simulink model "dk_luc"  (R2016a)
settings: Solver=ode45  StartTime=0.0  StopTime=322  RelTol=1e-3
settings Model: Creator=Trinh Hoang Minh  LastModifiedBy=Nam Nguyen
settings DataIOCC: LimitDataPoints=on  SaveFormat=Array  SignalLoggingSaveFormat=ModelDataLogs
settings OptimizationCC: ExpressionDepthLimit=2147483647
settings DebuggingCC: UnderspecifiedInitializationDetection=Classic  MergeDetectMultiDrivingBlocksExec=none  SolverPrmCheckMsg=warning  FcnCallInpInsideContextMsg=EnableAllAsWarning  StateNameClashWarn=warning
settings HardwareCC: ProdBitPerPointer=32  ProdLargestAtomicFloat=None  ProdIntDivRoundTo=Undefined  ProdEndianess=Unspecified  ProdWordSize=32  ProdHWDeviceType=32-bit Generic
settings ModelReferenceCC: PropagateSignalLabelsOutOfModel=off
settings ConfigComp: CovModelRefEnable=Off  CovSFcnEnable=off

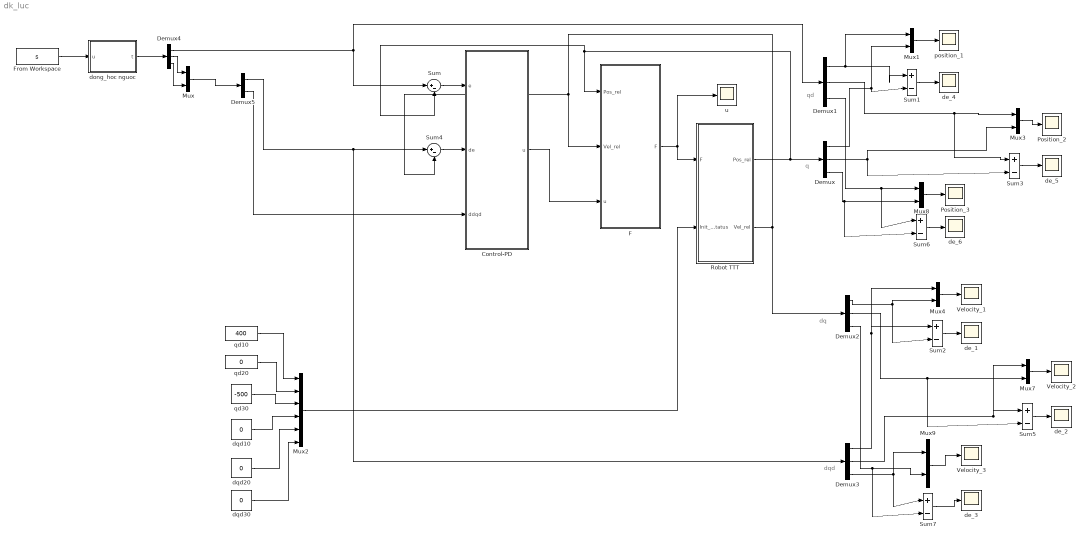
== system dk_luc ==
  note: q
  note: dq
  note: qd
  note: dqd
  Control-PD : Subsystem
  Demux{,1..4} (5 alike) : Demux  Outputs=3
  Demux5 : Demux  Outputs=2
  F : Subsystem
  From Workspace : FromWorkspace  VariableName=s  SampleTime=0.01
  Mux{,1,3..4,7..9} (7 alike) : Mux  Inputs=2
  Mux2 : Mux  Inputs=6
  Position_2 : Scope
  Position_3 : Scope
  "Robot TTT " : Subsystem
  Sum{,1..7} (8 alike) : Sum  Inputs=|+-
  Velocity_1 : Scope
  Velocity_2 : Scope
  Velocity_3 : Scope
  de_{1..6} (6 alike) : Scope
  dong_hoc nguoc : MATLAB Function  TreatAsAtomicUnit=on
  dqd10 : Constant  Value=0
  dqd20 : Constant  Value=0
  dqd30 : Constant  Value=0
  position_1 : Scope
  qd10 : Constant  Value=400
  qd20 : Constant  Value=0
  qd30 : Constant  Value=-500
  u : Scope
  wires:
  "Robot TTT "/2(Vel_rel) -> Demux2/1, Sum4/2, F/2(Vel_rel)
  Mux2/1 -> "Robot TTT "/2(Init_status)
  Control-PD/1(u) -> F/3(u)
  F/1(F) -> "Robot TTT "/1(F), u/1
  Mux1/1 -> position_1/1
  Mux3/1 -> Position_2/1
  "Robot TTT "/1(Pos_rel) -> Demux/1, Sum/2, F/1(Pos_rel)
  Demux1/1 -> Sum1/1, Mux1/1
  Demux1/2 -> Sum3/1, Mux3/1
  Demux/1 -> Sum1/2, Mux1/2
  Demux/2 -> Mux3/2, Sum3/2
  qd10/1 -> Mux2/1
  qd20/1 -> Mux2/2
  dqd10/1 -> Mux2/4
  Demux5/2 -> Control-PD/3(ddqd)
  Sum4/1 -> Control-PD/2(de)
  Demux5/1 -> Sum4/1, Demux3/1
  Sum/1 -> Control-PD/1(e)
  qd30/1 -> Mux2/3
  Mux4/1 -> Velocity_1/1
  Demux2/1 -> Mux4/2, Sum2/2
  Demux3/1 -> Sum2/1, Mux4/1
  Sum2/1 -> de_1/1
  Sum5/1 -> de_2/1
  Demux3/2 -> Mux7/1, Sum5/1
  Demux2/2 -> Sum5/2, Mux7/2
  Mux7/1 -> Velocity_2/1
  dqd20/1 -> Mux2/5
  dqd30/1 -> Mux2/6
  Demux1/3 -> Sum6/1, Mux8/1
  Demux/3 -> Sum6/2, Mux8/2
  Mux8/1 -> Position_3/1
  Demux2/3 -> Mux9/2, Sum7/2
  Mux9/1 -> Velocity_3/1
  Demux3/3 -> Mux9/1, Sum7/1
  Sum7/1 -> de_3/1
  Demux4/1 -> Sum/1, Demux1/1
  From Workspace/1 -> dong_hoc nguoc/1(u)
  Sum1/1 -> de_4/1
  Sum3/1 -> de_5/1
  dong_hoc nguoc/1(t) -> Demux4/1
  Sum6/1 -> de_6/1
  Demux4/2 -> Mux/1
  Demux4/3 -> Mux/2
  Mux/1 -> Demux5/1

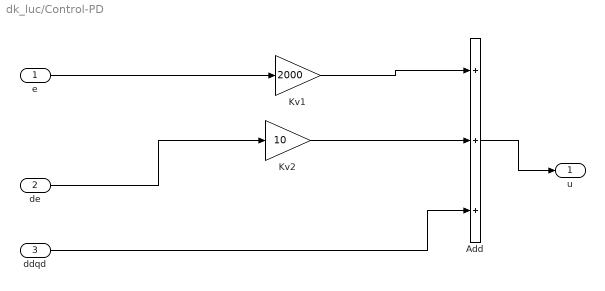
== system dk_luc/Control-PD ==
  e : Inport
  de : Inport  Port=2
  ddqd : Inport  Port=3
  Add : Sum  Inputs=+++
  Kv1 : Gain  Gain=2000
  Kv2 : Gain  Gain=10
  u : Outport
  wires:
  e/1 -> Kv1/1
  Kv1/1 -> Add/1
  de/1 -> Kv2/1
  Kv2/1 -> Add/2
  ddqd/1 -> Add/3
  Add/1 -> u/1

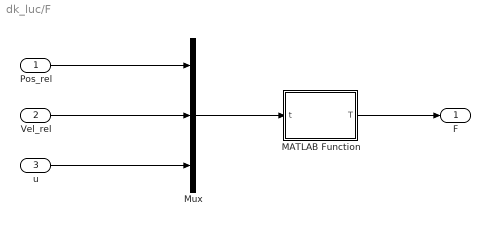
== system dk_luc/F ==
  Pos_rel : Inport
  Vel_rel : Inport  Port=2
  u : Inport  Port=3
  MATLAB Function : MATLAB Function  TreatAsAtomicUnit=on
  Mux : Mux  Inputs=3
  F : Outport
  wires:
  Pos_rel/1 -> Mux/1
  Vel_rel/1 -> Mux/2
  u/1 -> Mux/3
  Mux/1 -> MATLAB Function/1(t)
  MATLAB Function/1(T) -> F/1

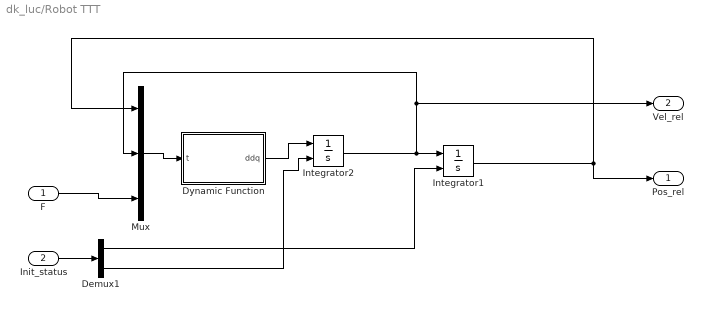
== system dk_luc/Robot TTT  ==
  F : Inport
  Init_status : Inport  Port=2
  Demux1 : Demux  Outputs=2
  Dynamic Function : MATLAB Function  TreatAsAtomicUnit=on
  Integrator1 : Integrator  InitialConditionSource=external
  Integrator2 : Integrator  InitialConditionSource=external
  Mux : Mux  Inputs=3
  Pos_rel : Outport
  Vel_rel : Outport  Port=2
  wires:
  Dynamic Function/1(ddq) -> Integrator2/1
  Init_status/1 -> Demux1/1
  Mux/1 -> Dynamic Function/1(t)
  Integrator1/1 -> Mux/1, Pos_rel/1
  F/1 -> Mux/3
  Demux1/2 -> Integrator2/2
  Integrator2/1 -> Mux/2, Vel_rel/1, Integrator1/1
  Demux1/1 -> Integrator1/2

== matlab function dk_luc/F/MATLAB Function ==
  data: t input; T output
function T = InverseModel(t)
m1 = 25.24; m2 = 44.4; m3 = 2.5;
g = 9.81;
Fx=22; Fy=2; Fz=10;
% vector toa do suy rong (toa do khop)
q = t(1:3);
% vector dao ham cac toa do suy rong (toa do khop)
dq = t(4:6);
% vector luc suy rong ung voi cac toa do suy rong (toa do khop)
u = t(7:9).';
% Ma tran khoi luong
m11=m1+m2+m3; 
m12 = 0;
m13=0;
m21 = m12;
m22 = m3+m2;
m23 =0;
m31=m13;
m32=m23;
m33=m3;
M = [m11,m12,m13;m21,m22,m23;m31,m32,m33];
% Luc qun tinh coriolis  va qun tinh li tam
Psi=[0;0;0];
% Luc suy rong cua cac luc co the
G = [0;g*(m2+m3); 0];
% Luc suy rong cua cac luc khong the
Q=[Fz;Fx;-Fy];
% Luc dan dong tai cac khop
T = M*[u(1);u(2);u(3)]+Psi+G+Q

== matlab function dk_luc/Robot TTT /Dynamic Function ==
  data: t input; ddq output
function ddq = RobotDynamic(t)
% cac tham so dong hoc, dong luc hoc
m1 = 25.24; m2 = 44.4; m3 = 2.5;
g = 9.81;

Fx=20; Fy=20; Fz=10;

% vector toa do suy rong (toa do khop)
q = t(1:3);
% vector dao ham cac toa do suy rong (toa do khop)
dq = t(4:6);
% vector luc suy rong ung voi cac toa do suy rong (toa do khop)
U = t(7:9).';
%load = t(10);
%m3 = load + m3;

% Ma tran khoi luong
m11=m1+m2+m3; 
m12 = 0;
m13=0;

m21 = m12;
m22 = m3+m2;
m23 =0;

m31=m13;
m32=m23;
m33=m3;

M = [m11,m12,m13;m21,m22,m23;m31,m32,m33];

% Luc qun tinh coriolis  va qun tinh li tam


Psi=[0;0;0];

% Luc suy rong cua cac luc co the
G = [0;g*(m2+m3); 0];

% Luc suy rong cua cac luc khong the
%Q1=0.2*dq(1);
%Q2=0.2*dq(2);

Q=[Fz;Fx;-Fy];

% Gia toc suy rong 
ddq = inv(M)*([U(1);U(2);U(3)]-Psi-G-Q);

== matlab function dk_luc/dong_hoc nguoc ==
  data: u input; t output
function t = fcn(u)
%#codegen
x=u(1);
y=u(2);
z=u(3);
vx=u(4);
vy=u(5);
vz=u(6);
ax=u(7);
ay=u(8);
az=u(9)
d1=60;
d2=360;
d3=620;
a3=110;
%vi tri
t1=z-d1;
t2=-x+d2-a3;
t3=-y-d3;
%van toc
t1_dot=vz;
t2_dot=-vx;
t3_dot=-vy;
%gia  toc
t1_2dot=az;
t2_2dot=-ax;
t3_2dot=-ay;
t=[t1 t2 t3 t1_dot t2_dot t3_dot t1_2dot t2_2dot t3_2dot]
